simulink model "c28x_CAN_acceptance_filtering"  (R2021b)
settings: Solver=FixedStepDiscrete  StartTime=0.0  StopTime=Inf  RelTol=1e-3  EnableMultiTasking=on
libraries: c280xlib x8, c2000lib x1, demo_controls x1, canmsglib x1
settings Model: ExtModeTrigDuration=8  Creator=The MathWorks, Inc.  LastModifiedBy=The MathWorks, Inc.
settings OptimizationCC: DefaultUnderspecifiedDataType=single  EnhancedBackFolding=on  PassReuseOutputArgsAs=Individual arguments  MaxStackSize=1024  OptimizeBlockOrder=speed  DifferentSizesBufferReuse=on  OptimizationCustomize=off  DenormalBehavior=FlushToZero  EfficientTunableParamExpr=on
settings DebuggingCC: ParameterTunabilityLossMsg=error
settings HardwareCC: ProdBitPerChar=16  ProdBitPerInt=16  ProdBitPerPointer=32  ProdBitPerSizeT=32  ProdBitPerPtrDiffT=32  ProdLargestAtomicInteger=Integer  ProdLargestAtomicFloat=None  ProdWordSize=16  ProdLongLongMode=on  ProdHWDeviceType=Texas Instruments->C2000
settings SFSimCC: MATLABDynamicMemAlloc=off
settings RTWCC: Description=Embedded Coder  SystemTargetFile=ert.tlc  HardwareBoard=TI Piccolo F28069M LaunchPad  TemplateMakefile=ert_default_tmf  Toolchain=Texas Instruments Code Composer Studio (C2000)  BuildConfiguration=Debug
settings CodeAppCC: ForceParamTrailComments=on  IgnoreCustomStorageClasses=off  OperatorAnnotations=on  SimulinkDataObjDesc=on  SFDataObjDesc=on  InsertBlockDesc=on
settings ERTTargetCC: CodeReplacementLibrary=TI C28x  ExtModeTransport=3  ExtModeStaticAlloc=on  ExtModeStaticAllocSize=10000

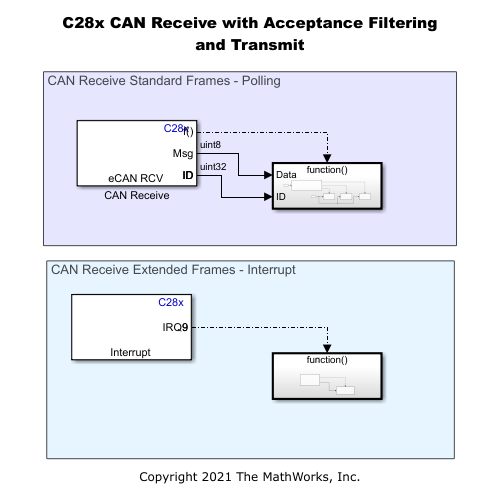
[thumbnail: Simulink's stored preview of the top-level diagram]
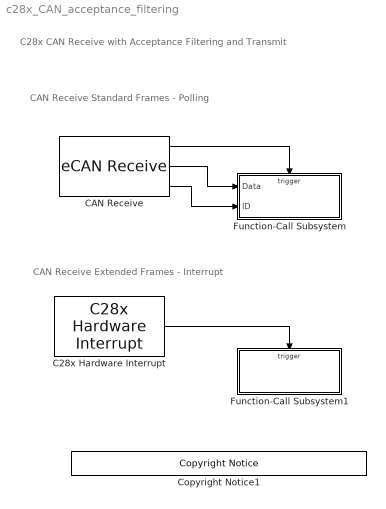
== system c28x_CAN_acceptance_filtering ==
  note: C28x CAN Receive with Acceptance Filtering
      | and Transmit
  note: CAN Receive Extended Frames - Interrupt
  note: CAN Receive Standard Frames - Polling
  C28x Hardware Interrupt : c2000lib/Scheduling/C28x Hardware Interrupt  irqnumbers=[9]  pienumbers=[6]  irqpriorities=[30]  irqpreempts=[1]  showinput=off  dspchiptype=C280X
      settings: SourceProductBaseCode=TIC2000
  CAN Receive : c280xlib/eCAN Receive  chipFamily=C280x  useModule=eCAN_A  mailboxNo=2  messageID=hex2dec('0x0000001')  messageType=Standard (11-bit identifier)  enableAcceptanceFiltering=on  messageIDMask=hex2dec('0x00000007')  sampleTime=0.001  dataType=uint8  outputAction=Reset all fields to zero  initValue=255  outputMessageID=on  outputMessageLength=off  outputMessageTimeStamp=off  postInterrupt=off  interruptLine=0
      settings: SourceProductBaseCode=TIC2000
  Copyright Notice1 : demo_controls/Copyright Notice  year=2021  prod=tic2000
      settings: SourceProductBaseCode=ME
  Function-Call Subsystem : Subsystem  TreatAsAtomicUnit=on
  Function-Call Subsystem1 : Subsystem  TreatAsAtomicUnit=on
  wires:
  C28x Hardware Interrupt/1 -> Function-Call Subsystem1/Trigger
  CAN Receive/1 -> Function-Call Subsystem/Trigger
  CAN Receive/2 -> Function-Call Subsystem/1(Data)
  CAN Receive/3 -> Function-Call Subsystem/2(ID)

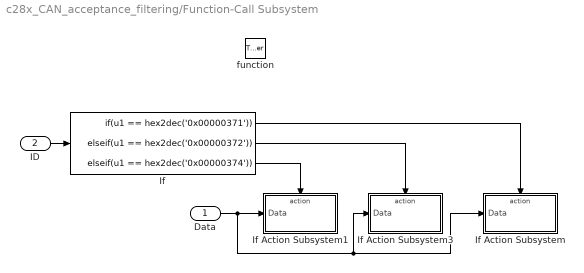
== system c28x_CAN_acceptance_filtering/Function-Call Subsystem ==
  Data : Inport
  ID : Inport  Port=2
  function : TriggerPort  TriggerType=function-call  VariantControl=(inherit)
  If : If  IfExpression=u1 == hex2dec('0x00000371')  ElseIfExpressions=u1 == hex2dec('0x00000372'), u1 == hex2dec('0x00000374')  ShowElse=off
  If Action Subsystem : Subsystem  TreatAsAtomicUnit=on
  If Action Subsystem1 : Subsystem  TreatAsAtomicUnit=on
  If Action Subsystem3 : Subsystem  TreatAsAtomicUnit=on
  wires:
  ID/1 -> If/1
  If/1 -> If Action Subsystem/Action
  If/2 -> If Action Subsystem3/Action
  If/3 -> If Action Subsystem1/Action
  Data/1 -> If Action Subsystem/1(Data), If Action Subsystem3/1(Data), If Action Subsystem1/1(Data)

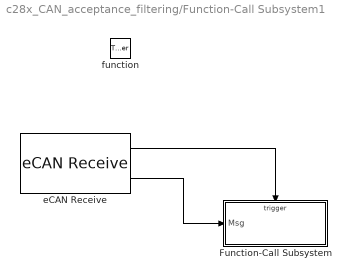
== system c28x_CAN_acceptance_filtering/Function-Call Subsystem1 ==
  function : TriggerPort  TriggerType=function-call  VariantControl=(inherit)
  Function-Call Subsystem : Subsystem  TreatAsAtomicUnit=on
  eCAN Receive : c280xlib/eCAN Receive  chipFamily=C280x  useModule=eCAN_A  mailboxNo=3  messageID=hex2dec('0x00000003')  messageType=Extended (29-bit identifier)  enableAcceptanceFiltering=on  messageIDMask=hex2dec('0x00000007')  sampleTime=-1  dataType=CAN_MESSAGE_TYPE  outputAction=Output last received values  initValue=255  outputMessageID=off  outputMessageLength=off  outputMessageTimeStamp=off  postInterrupt=on  interruptLine=1
      settings: SourceProductBaseCode=TIC2000
  wires:
  eCAN Receive/1 -> Function-Call Subsystem/Trigger
  eCAN Receive/2 -> Function-Call Subsystem/1(Msg)

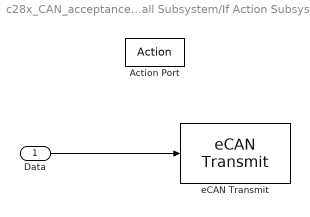
== system c28x_CAN_acceptance_filtering/Function-Call Subsystem/If Action Subsystem ==
  Data : Inport
  Action Port : ActionPort  ActionPortLabel=if(u1 == hex2dec('0x00000371'))
  eCAN Transmit : c280xlib/eCAN Transmit  chipFamily=C280x  useModule=eCAN_A  mailboxNo=1  messageID=hex2dec('0x00000001')  messageType=Standard (11-bit identifier)  enableBlockingMode=off  postInterrupt=off  interruptLine=0
      settings: SourceProductBaseCode=TIC2000
  wires:
  Data/1 -> eCAN Transmit/1

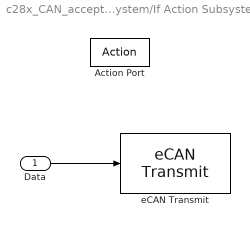
== system c28x_CAN_acceptance_filtering/Function-Call Subsystem/If Action Subsystem1 ==
  Data : Inport
  Action Port : ActionPort  ActionPortLabel=elseif( u1 == hex2dec('0x00000374'))
  eCAN Transmit : c280xlib/eCAN Transmit  chipFamily=C280x  useModule=eCAN_A  mailboxNo=1  messageID=hex2dec('0x00000004')  messageType=Standard (11-bit identifier)  enableBlockingMode=off  postInterrupt=off  interruptLine=0
      settings: SourceProductBaseCode=TIC2000
  wires:
  Data/1 -> eCAN Transmit/1

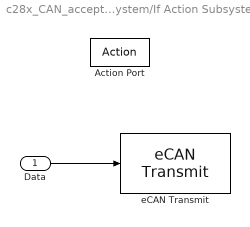
== system c28x_CAN_acceptance_filtering/Function-Call Subsystem/If Action Subsystem3 ==
  Data : Inport
  Action Port : ActionPort  ActionPortLabel=elseif(u1 == hex2dec('0x00000372'))
  eCAN Transmit : c280xlib/eCAN Transmit  chipFamily=C280x  useModule=eCAN_A  mailboxNo=1  messageID=hex2dec('0x00000002')  messageType=Standard (11-bit identifier)  enableBlockingMode=off  postInterrupt=off  interruptLine=0
      settings: SourceProductBaseCode=TIC2000
  wires:
  Data/1 -> eCAN Transmit/1

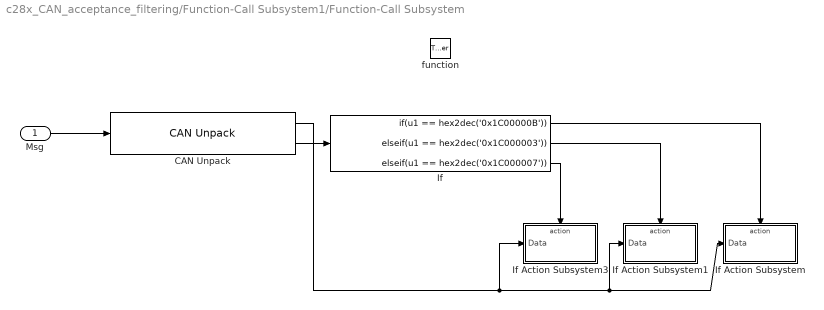
== system c28x_CAN_acceptance_filtering/Function-Call Subsystem1/Function-Call Subsystem ==
  Msg : Inport
  function : TriggerPort  TriggerType=function-call  VariantControl=(inherit)
  CAN Unpack : canmsglib/CAN Unpack  MsgList=(none)  MsgName=CAN Msg  MsgIDType=Extended (29-bit identifier)  MsgIdentifier=-1  MsgLength=8  SignalInfo={}  IDPort=on  TimestampPort=off  ErrorPort=off  RemotePort=off  LengthPort=off  StatusPort=off  ApplyMinMax=off
      settings: SourceProductBaseCode=ME,XP,VN  DataFormat=raw data
  If : If  IfExpression=u1 == hex2dec('0x1C00000B')  ElseIfExpressions=u1 == hex2dec('0x1C000003'),u1 == hex2dec('0x1C000007')  ShowElse=off
  If Action Subsystem : Subsystem  TreatAsAtomicUnit=on
  If Action Subsystem1 : Subsystem  TreatAsAtomicUnit=on
  If Action Subsystem3 : Subsystem  TreatAsAtomicUnit=on
  wires:
  Msg/1 -> CAN Unpack/1
  CAN Unpack/2 -> If/1
  If/1 -> If Action Subsystem/Action
  CAN Unpack/1 -> If Action Subsystem3/1(Data), If Action Subsystem1/1(Data), If Action Subsystem/1(Data)
  If/3 -> If Action Subsystem3/Action
  If/2 -> If Action Subsystem1/Action

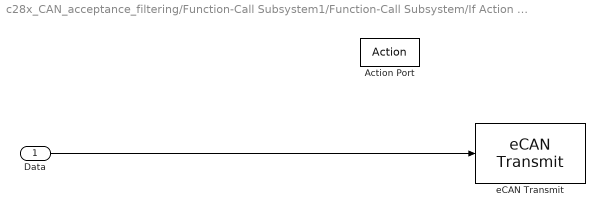
== system c28x_CAN_acceptance_filtering/Function-Call Subsystem1/Function-Call Subsystem/If Action Subsystem ==
  Data : Inport
  Action Port : ActionPort  ActionPortLabel=if(u1 == hex2dec('0x1C00000B'))
  eCAN Transmit : c280xlib/eCAN Transmit  chipFamily=C280x  useModule=eCAN_A  mailboxNo=1  messageID=hex2dec('0x0000000B')  messageType=Extended (29-bit identifier)  enableBlockingMode=off  postInterrupt=off  interruptLine=0
      settings: SourceProductBaseCode=TIC2000
  wires:
  Data/1 -> eCAN Transmit/1

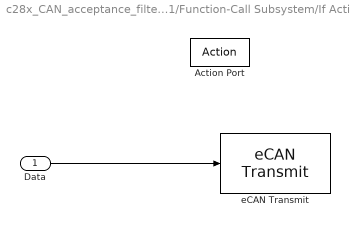
== system c28x_CAN_acceptance_filtering/Function-Call Subsystem1/Function-Call Subsystem/If Action Subsystem1 ==
  Data : Inport
  Action Port : ActionPort  ActionPortLabel=elseif(u1 == hex2dec('0x1C000003'))
  eCAN Transmit : c280xlib/eCAN Transmit  chipFamily=C280x  useModule=eCAN_A  mailboxNo=1  messageID=hex2dec('0x00000003')  messageType=Extended (29-bit identifier)  enableBlockingMode=off  postInterrupt=off  interruptLine=0
      settings: SourceProductBaseCode=TIC2000
  wires:
  Data/1 -> eCAN Transmit/1

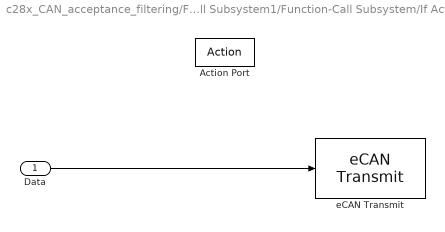
== system c28x_CAN_acceptance_filtering/Function-Call Subsystem1/Function-Call Subsystem/If Action Subsystem3 ==
  Data : Inport
  Action Port : ActionPort  ActionPortLabel=elseif(u1 == hex2dec('0x1C000007'))
  eCAN Transmit : c280xlib/eCAN Transmit  chipFamily=C280x  useModule=eCAN_A  mailboxNo=1  messageID=hex2dec('0x00000007')  messageType=Extended (29-bit identifier)  enableBlockingMode=off  postInterrupt=off  interruptLine=0
      settings: SourceProductBaseCode=TIC2000
  wires:
  Data/1 -> eCAN Transmit/1
